simulink model "robot_simplified"  (R2021b)
settings: Solver=VariableStepAuto  StartTime=0.0  StopTime=11  RelTol=1e-3
model workspace: external: MATLAB File C:\Users\victo\Documents\MATLAB\CAD\STEP\ssl-robot\robot_simplified_DataFile.m (data not in the file)
values from neighbouring files (symbols this model uses):
  control =     [robot_simplified_DataFile.mat]
  g = 9.80665    [robot_simplified_DataFile.m]    (also in robot_simplified_parameters.m = -9.80665)
undefined symbols (not defined in the file or in its folder): DiscIntNeverNeededParam, field, kinematics, SamplingTime, smiData, tire, tkd, tki, tkp, wheel, X, Y, Z
libraries: sm_lib x722, nesl_utility x23, simulink x5, slpidlib x4, cstblocks x4, SignalEditorBlockLib x1, eeBldcCurrentController x1
(part 1 of 8)
settings Model: Creator=victo  LastModifiedBy=victo

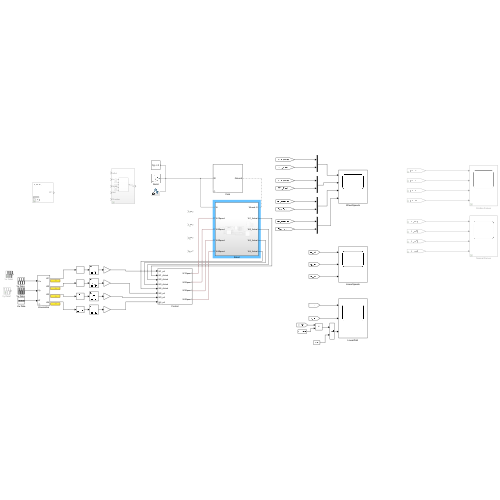
[thumbnail: Simulink's stored preview of the top-level diagram]
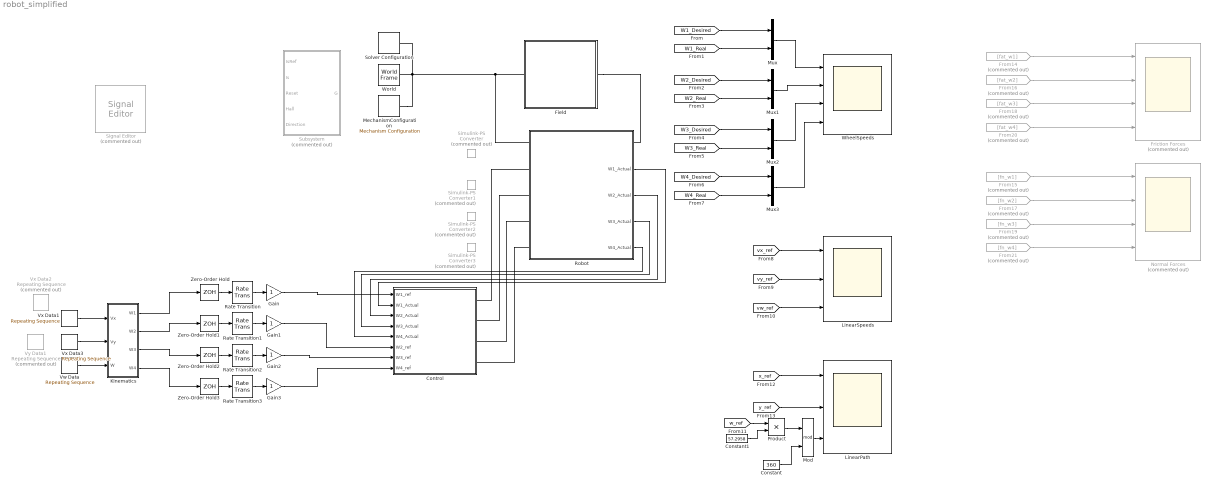
== system robot_simplified ==
  Constant : Constant  Value=360
  Constant1 : Constant  Value=57.2958
  Control : Subsystem  mask{T=SamplingTime, Kp=control.Kp, Ki=control.Ki, Ts=control.tf.Ts, df=control.tf.df, dm=control.tf.dm, FF=control.ff}
      mask prompts: T "Sampling Time"; Kp "Proportional"; Ki "Integral"
      mask DialogControl ControlParameters Prompt: Control Parameters
  Field : Subsystem  mask{fieldWidth=field.Width, fieldHeight=field.Height, fieldColor=field.Color}
      mask prompts: fieldWidth "Width(mm)"; fieldHeight "Height (mm)"; fieldColor "Color"
      mask DialogControl TabField Prompt: Field
  Friction Forces : Scope  Commented=on  NumInputPorts=4
  From14 : From  Commented=on  GotoTag=fat_w1
  From15 : From  Commented=on  GotoTag=fn_w1
  From16 : From  Commented=on  GotoTag=fat_w2
  From17 : From  Commented=on  GotoTag=fn_w2
  From18 : From  Commented=on  GotoTag=fat_w3
  From19 : From  Commented=on  GotoTag=fn_w3
  From20 : From  Commented=on  GotoTag=fat_w4
  From21 : From  Commented=on  GotoTag=fn_w4
  Gain{,1..3} (4 alike) : Gain
  Kinematics : Subsystem  mask{KinematicMatrix=kinematics.prod2}
      mask prompts: KinematicMatrix "Kinematics Function"
      mask DialogControl ParameterGroupVar0 Prompt: Kinematics Parameters
  LinearPath : Scope  NumInputPorts=3
  LinearSpeeds : Scope  NumInputPorts=3
  MechanismConfiguration : sm_lib/Utilities/Mechanism Configuration  UniformGravity=Constant  GravityVector="[0  0 -g]"  GravityUnits=m/s^2  LinearizationDelta=0.001  JointModeTransitionNonlinearIterations=2
  Mod : Math  Operator=mod  SaturateOnIntegerOverflow=on
  Mux{,1..3} (4 alike) : Mux  Inputs=2
  Normal Forces : Scope  Commented=on  NumInputPorts=4
  Product : Product
  Rate Transition : RateTransition  OutPortSampleTimeOpt=Inherit  OutPortSampleTime=0.002
  Rate Transition1 : RateTransition  OutPortSampleTimeOpt=Inherit  OutPortSampleTime=0.002
  Rate Transition2 : RateTransition  OutPortSampleTimeOpt=Inherit  OutPortSampleTime=0.01
  Rate Transition3 : RateTransition  OutPortSampleTimeOpt=Inherit  OutPortSampleTime=0.01
  Robot : Subsystem
      settings: PortSchema="{\"entries\":[{\"content\":{\"sides\":[{\"content\":{\"connectorIds\":[\"LConn1\",\"LConn2\",\"LConn3\",\"LConn4\",\"LConn5\"]},\"type\":\"ConnectorPlacement.EquallySpacedRectSide\",\"uuid\":\"253f09d1-5eeb-4b26-8135-d2db322c5f85\"},{\"content\":{\"connectorIds\":[\"RConn1\",\"Out1\",\"Out2\",\"Out3\",\"Out4\"],\"side\":\"RIGHT\"},\"type\":\"ConnectorPlacement.EquallySpacedRectSide\",\"uuid\":\"5e48723f-c100-4ab2-897b-63b213ce7996\"},{\"content\":{\"connectorIds\":[],\"side\":\"TOP\"},\"type\":\"ConnectorPlacement.EquallySpacedRectSide\",\"uuid\":\"88c9750e-929f-48a2-b612-d7f74cbee2f8\"}]},\"type\":\"ConnectorPlacement.EquallySpacedConnector\",\"uuid\":\"41f69800-7732-438a-91c0-e5f9fc926441\"}],\"packageUris\":[\"http://schema.mathworks.com/mf0/Connector/R2020b\"],\"version\":\"1.0\"}"
  Signal Editor : SignalEditorBlockLib/Signal Editor  Commented=on  FileName=Control_signals.mat  ActiveScenario=Scenario  ActiveSignal=W1  IsBus=off  OutputBusObjectStr=Bus: BusObject  SampleTime=0  ZeroCross=off  OutputAfterFinalValue=Holding final value  Unit=inherit  PreserveSignalName=on
  Simulink-PS Converter{,1..3} (4 alike) : nesl_utility/Simulink-PS Converter  Commented=on  PhysicalDomain=network_engine_domain  SubClassName=ps_input  LeftPortType=input  RightPortType=output  PseudoPeriodic=off  Frequencies=[]  NoiseDistribution=none  NoiseParameters=[]  Unit=1  AffineConversion=off  FilteringAndDerivatives=filter  SimscapeFilterOrder=2  InputFilterTimeConstant=0.001  UdotUserProvided=0
      settings: SourceProductBaseCode=PW,SS
  Solver Configuration : nesl_utility/Solver Configuration  PhysicalDomain=network_engine_domain  SubClassName=solver  LeftPortType=input  RightPortType=generic  Tones=[]  Harmonics=[]  SimulateNoise=off  Profile=off  UseLocalSampling=off  EnableSwitchedLinearOptims=on  FrequencyDomain=off  UseCCode=off  RelTol=0.001  AbsTol=1e-06  MinStep=1e-09  ToWorkspace=off  RevertToSquareIcSolve=off  NumHomotopyIterations=100  PhasorMode=off  PhasorModeNumHarmonics=1  DoDC=off  ResidualTolerance=1e-09  UseLocalSolver=off  LocalSolverChoice=NE_BACKWARD_EULER_ADVANCER  LocalSolverSampleTime=0.001  DoFixedCost=off  MaxNonlinIter=3  MaxModeIter=2  ComputeImpulses=off  ImpulseIterations=2  LinearAlgebra=Sparse  EquationFormulation=NE_TIME_EF  DelaysMemoryBudget=1024  AutomaticFiltering=on  FilteringTimeConstant=0.001  PartitionStorageMethod=AS_NEEDED  PartitionMemoryBudget=1024  PartitionMethod=ROBUST
      settings: SourceProductBaseCode=PW,SS
  Subsystem : Subsystem  Commented=on
  Vw Data : simulink/Sources/Repeating Sequence  rep_seq_t=[0 2 3 9.3 9.7 11]  rep_seq_y=[0 0 0 0 0 0]
  Vx Data1 : simulink/Sources/Repeating Sequence  rep_seq_t=[0 0.2 1 1.6 2.4 3.2 3.8 4.3 4.5 5.3 6 6.6 7 7.8 8.4 8.9 9.1 9.9 10.5 11]  rep_seq_y=[0 0 -0.75 0 0 0 0 0 0 0.75 0.75 0 0 0 0 0 0 -0.75 0 0]
  Vx Data2 : simulink/Sources/Repeating Sequence  Commented=on  rep_seq_t="[0 4.7  5.7 9.2 9.7 14.7 15.7 19.2 19.7 20]"  rep_seq_y=[0 0 -0.75 -0.75 0 0 0.75 0.75 0 0]
  Vx Data3 : simulink/Sources/Repeating Sequence  rep_seq_t=[0 0.2 1 1.6 2.3 3 3.8 4.1 4.3 4.5 5.3 6 6.6 6.7 7.4 8.2 8.5 8.9 9.1 9.9 10.5 11]  rep_seq_y=[0 0 -0.75 0 0 0.75 0.75 0 0 0 -0.75 -0.75 0 0 0.75 0.75 0 0 0 -0.75 0 0]
  Vy Data1 : simulink/Sources/Repeating Sequence  Commented=on  rep_seq_t=[0 0.2 1.2 3.7 4.2 10.2 11.2 13.7 14.2 20]  rep_seq_y=[0 0 0.75 0.75 0 0 -0.75 -0.75 0 0]
  WheelSpeeds : Scope  NumInputPorts=4
  World : sm_lib/Frames and Transforms/World Frame
  Zero-Order Hold{,1..3} (4 alike) : ZeroOrderHold  SampleTime=0.002
  wires:
  Mux/1 -> WheelSpeeds/1
  Robot/2(W2_Actual) -> Control/3(W2_Actual)
  Robot/3(W3_Actual) -> Control/4(W3_Actual)
  Robot/4(W4_Actual) -> Control/5(W4_Actual)
  [W2_Desired] -> Mux1/1
  [W2_Real] -> Mux1/2
  [W3_Desired] -> Mux2/1
  [W3_Real] -> Mux2/2
  [W4_Desired] -> Mux3/1
  [W4_Real] -> Mux3/2
  Rate Transition/1 -> Gain/1
  Zero-Order Hold/1 -> Rate Transition/1
  Zero-Order Hold1/1 -> Rate Transition1/1
  Rate Transition1/1 -> Gain1/1
  Zero-Order Hold2/1 -> Rate Transition2/1
  Rate Transition2/1 -> Gain2/1
  Zero-Order Hold3/1 -> Rate Transition3/1
  Rate Transition3/1 -> Gain3/1
  Gain/1 -> Control/1(W1_ref)
  Robot/1(W1_Actual) -> Control/2(W1_Actual)
  Gain1/1 -> Control/6(W2_ref)
  Gain2/1 -> Control/7(W3_ref)
  Gain3/1 -> Control/8(W4_ref)
  [W1_Real] -> Mux/2
  [W1_Desired] -> Mux/1
  Mux1/1 -> WheelSpeeds/2
  Mux2/1 -> WheelSpeeds/3
  Mux3/1 -> WheelSpeeds/4
  [vx_ref] -> LinearSpeeds/1
  [vy_ref] -> LinearSpeeds/2
  [vw_ref] -> LinearSpeeds/3
  [x_ref] -> LinearPath/1
  [y_ref] -> LinearPath/2
  Constant/1 -> Mod/2
  Mod/1 -> LinearPath/3
  [w_ref] -> Product/1
  Constant1/1 -> Product/2
  Product/1 -> Mod/1
  Vw Data/1 -> Kinematics/3(W)
  Kinematics/4(W4) -> Zero-Order Hold3/1
  Kinematics/1(W1) -> Zero-Order Hold/1
  Kinematics/2(W2) -> Zero-Order Hold1/1
  Kinematics/3(W3) -> Zero-Order Hold2/1
  Vx Data3/1 -> Kinematics/2(Vy)
  Vx Data1/1 -> Kinematics/1(Vx)
  From14/1 -> Friction Forces/1
  From18/1 -> Friction Forces/3
  From17/1 -> Normal Forces/2
  From20/1 -> Friction Forces/4
  From19/1 -> Normal Forces/3
  From16/1 -> Friction Forces/2
  From21/1 -> Normal Forces/4
  From15/1 -> Normal Forces/1
  connections:
  MechanismConfiguration/RConn1 -- Field/LConn1 -- Robot/LConn1 -- Solver Configuration/RConn1 -- World/RConn1
  Field/RConn1 -- Robot/RConn1
  Robot/LConn2 -- Control/RConn1
  Robot/LConn3 -- Control/RConn2
  Robot/LConn4 -- Control/RConn3
  Robot/LConn5 -- Control/RConn4

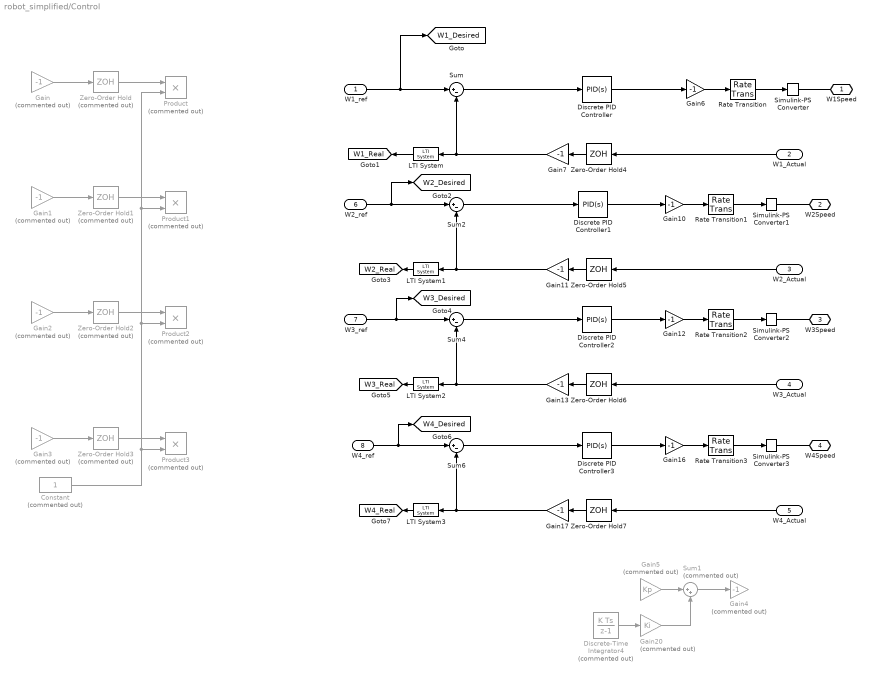
== system robot_simplified/Control ==
  W1_ref : Inport
  W1_Actual : Inport  Port=2
  W2_Actual : Inport  Port=3
  W3_Actual : Inport  Port=4
  W4_Actual : Inport  Port=5
  W2_ref : Inport  Port=6
  W3_ref : Inport  Port=7
  W4_ref : Inport  Port=8
  Constant : Constant  Commented=on
  Discrete PID Controller : slpidlib/PID Controller  Controller=PID  Form=Parallel  TimeDomain=Continuous-time  UseExternalTs=off  SampleTime=-1  IntegratorMethod=Forward Euler  FilterMethod=Forward Euler  ControllerParametersSource=internal  P=tkp  I=tki  D=tkd  UseFilter=on  N=8276.77127710328  TunerSelectOption=Transfer Function Based (PID Tuner App)  InitialConditionSource=internal  InitialConditionForIntegrator=0  InitialConditionForFilter=0  DifferentiatorICPrevScaledInput=0  ExternalReset=none  TrackingMode=off  Kt=1  LimitOutput=off  SatLimitsSource=internal  UpperSaturationLimit=2527  LowerSaturationLimit=-2527  LinearizeAsGain=off  AntiWindupMode=clamping  Kb=1  POutMin=[]  POutMax=[]  IOutMin=[]  IOutMax=[]  DOutMin=[]  DOutMax=[]  NOutMin=[]  NOutMax=[]  SumOutMin=[]  SumOutMax=[]  SaturationOutMin=[]  SaturationOutMax=[]  PParamMin=[]  PParamMax=[]  IParamMin=[]  IParamMax=[]  DParamMin=[]  DParamMax=[]  NParamMin=[]  NParamMax=[]  KbParamMin=[]  KbParamMax=[]  KtParamMin=[]  KtParamMax=[]  KbOutMin=[]  KbOutMax=[]  KtOutMin=[]  KtOutMax=[]  IntegratorOutMin=[]  IntegratorOutMax=[]  FilterOutMin=[]  FilterOutMax=[]  SumI1OutMin=[]  SumI1OutMax=[]  SumI2OutMin=[]  SumI2OutMax=[]  SumI3OutMin=[]  SumI3OutMax=[]  SumI4OutMin=[]  SumI4OutMax=[]  SumDOutMin=[]  SumDOutMax=[]  DifferentiatorOutMin=[]  DifferentiatorOutMax=[]  FilterDiffOutCoefMin=[]  FilterDiffOutCoefMax=[]  ReciprocalOutMin=[]  ReciprocalOutMax=[]  SumDenOutMin=[]  SumDenOutMax=[]  SumNumOutMin=[]  SumNumOutMax=[]  DivideOutMin=[]  DivideOutMax=[]  UdiffTsProdOutMin=[]  UdiffTsProdOutMax=[]  NTsProdOutMin=[]  NTsProdOutMax=[]  UintegralTsProdOutMin=[]  UintegralTsProdOutMax=[]  UngainTsProdOutMin=[]  UngainTsProdOutMax=[]  IntegratorContinuousStateAttributes=''  IntegratorStateMustResolveToSignalObject=off  IntegratorRTWStateStorageClass=Auto  FilterContinuousStateAttributes=''  FilterStateMustResolveToSignalObject=off  FilterRTWStateStorageClass=Auto  ParallelPVariant=InternalParameters  IdealPVariant=Disabled  IVariant=InternalParameters  DVariant=InternalParameters  IntegratorVariant=Continuous  SatVariant=Disabled  AWVariant=Passthrough  PCopyVariant=Disabled  TRVariant=Disabled  FdbkBlocksVariant=Forward  IdealPFdbkVariant=Disabled  SatFdbkVariant=Disabled  DerivativeFilterVariant=ContFilter  NVariant=InternalParameters  NCopyVariant=Disabled  FilterICVariant=InternalICsFilter  IntegratorICVariant=InternalICs  ExternalResetVariant=Disabled  TRSumVariant=Passthrough  SumFdbkVariant=Disabled  SumVariant=Sum_PID  TsampFilterVariant=InternalTs  TsampNgainVariant=Passthrough  TsampIntegralVariant=Passthrough  ExternalSaturationOutDataTypeStr=Inherit: Same as second input
  Discrete PID Controller1 : slpidlib/PID Controller  Controller=PID  Form=Parallel  TimeDomain=Continuous-time  UseExternalTs=off  SampleTime=0.01  IntegratorMethod=Forward Euler  FilterMethod=Forward Euler  ControllerParametersSource=internal  P=tkp  I=tki  D=tkd  UseFilter=on  N=7595.87594615657  TunerSelectOption=Transfer Function Based (PID Tuner App)  InitialConditionSource=internal  InitialConditionForIntegrator=0  InitialConditionForFilter=0  DifferentiatorICPrevScaledInput=0  ExternalReset=none  TrackingMode=off  Kt=1  LimitOutput=off  SatLimitsSource=internal  UpperSaturationLimit=2527  LowerSaturationLimit=-2527  LinearizeAsGain=off  AntiWindupMode=clamping  Kb=1  POutMin=[]  POutMax=[]  IOutMin=[]  IOutMax=[]  DOutMin=[]  DOutMax=[]  NOutMin=[]  NOutMax=[]  SumOutMin=[]  SumOutMax=[]  SaturationOutMin=[]  SaturationOutMax=[]  PParamMin=[]  PParamMax=[]  IParamMin=[]  IParamMax=[]  DParamMin=[]  DParamMax=[]  NParamMin=[]  NParamMax=[]  KbParamMin=[]  KbParamMax=[]  KtParamMin=[]  KtParamMax=[]  KbOutMin=[]  KbOutMax=[]  KtOutMin=[]  KtOutMax=[]  IntegratorOutMin=[]  IntegratorOutMax=[]  FilterOutMin=[]  FilterOutMax=[]  SumI1OutMin=[]  SumI1OutMax=[]  SumI2OutMin=[]  SumI2OutMax=[]  SumI3OutMin=[]  SumI3OutMax=[]  SumI4OutMin=[]  SumI4OutMax=[]  SumDOutMin=[]  SumDOutMax=[]  DifferentiatorOutMin=[]  DifferentiatorOutMax=[]  FilterDiffOutCoefMin=[]  FilterDiffOutCoefMax=[]  ReciprocalOutMin=[]  ReciprocalOutMax=[]  SumDenOutMin=[]  SumDenOutMax=[]  SumNumOutMin=[]  SumNumOutMax=[]  DivideOutMin=[]  DivideOutMax=[]  UdiffTsProdOutMin=[]  UdiffTsProdOutMax=[]  NTsProdOutMin=[]  NTsProdOutMax=[]  UintegralTsProdOutMin=[]  UintegralTsProdOutMax=[]  UngainTsProdOutMin=[]  UngainTsProdOutMax=[]  IntegratorContinuousStateAttributes=''  IntegratorStateMustResolveToSignalObject=off  IntegratorRTWStateStorageClass=Auto  FilterContinuousStateAttributes=''  FilterStateMustResolveToSignalObject=off  FilterRTWStateStorageClass=Auto  ParallelPVariant=InternalParameters  IdealPVariant=Disabled  IVariant=InternalParameters  DVariant=InternalParameters  IntegratorVariant=Continuous  SatVariant=Disabled  AWVariant=Passthrough  PCopyVariant=Disabled  TRVariant=Disabled  FdbkBlocksVariant=Forward  IdealPFdbkVariant=Disabled  SatFdbkVariant=Disabled  DerivativeFilterVariant=ContFilter  NVariant=InternalParameters  NCopyVariant=Disabled  FilterICVariant=InternalICsFilter  IntegratorICVariant=InternalICs  ExternalResetVariant=Disabled  TRSumVariant=Passthrough  SumFdbkVariant=Disabled  SumVariant=Sum_PID  TsampFilterVariant=InternalTs  TsampNgainVariant=Passthrough  TsampIntegralVariant=Passthrough  ExternalSaturationOutDataTypeStr=Inherit: Same as second input
  Discrete PID Controller2 : slpidlib/PID Controller  Controller=PID  Form=Parallel  TimeDomain=Continuous-time  UseExternalTs=off  SampleTime=0.01  IntegratorMethod=Forward Euler  FilterMethod=Forward Euler  ControllerParametersSource=internal  P=tkp  I=tki  D=tkd  UseFilter=on  N=7595.87594615657  TunerSelectOption=Transfer Function Based (PID Tuner App)  InitialConditionSource=internal  InitialConditionForIntegrator=0  InitialConditionForFilter=0  DifferentiatorICPrevScaledInput=0  ExternalReset=none  TrackingMode=off  Kt=1  LimitOutput=off  SatLimitsSource=internal  UpperSaturationLimit=2527  LowerSaturationLimit=-2527  LinearizeAsGain=off  AntiWindupMode=clamping  Kb=1  POutMin=[]  POutMax=[]  IOutMin=[]  IOutMax=[]  DOutMin=[]  DOutMax=[]  NOutMin=[]  NOutMax=[]  SumOutMin=[]  SumOutMax=[]  SaturationOutMin=[]  SaturationOutMax=[]  PParamMin=[]  PParamMax=[]  IParamMin=[]  IParamMax=[]  DParamMin=[]  DParamMax=[]  NParamMin=[]  NParamMax=[]  KbParamMin=[]  KbParamMax=[]  KtParamMin=[]  KtParamMax=[]  KbOutMin=[]  KbOutMax=[]  KtOutMin=[]  KtOutMax=[]  IntegratorOutMin=[]  IntegratorOutMax=[]  FilterOutMin=[]  FilterOutMax=[]  SumI1OutMin=[]  SumI1OutMax=[]  SumI2OutMin=[]  SumI2OutMax=[]  SumI3OutMin=[]  SumI3OutMax=[]  SumI4OutMin=[]  SumI4OutMax=[]  SumDOutMin=[]  SumDOutMax=[]  DifferentiatorOutMin=[]  DifferentiatorOutMax=[]  FilterDiffOutCoefMin=[]  FilterDiffOutCoefMax=[]  ReciprocalOutMin=[]  ReciprocalOutMax=[]  SumDenOutMin=[]  SumDenOutMax=[]  SumNumOutMin=[]  SumNumOutMax=[]  DivideOutMin=[]  DivideOutMax=[]  UdiffTsProdOutMin=[]  UdiffTsProdOutMax=[]  NTsProdOutMin=[]  NTsProdOutMax=[]  UintegralTsProdOutMin=[]  UintegralTsProdOutMax=[]  UngainTsProdOutMin=[]  UngainTsProdOutMax=[]  IntegratorContinuousStateAttributes=''  IntegratorStateMustResolveToSignalObject=off  IntegratorRTWStateStorageClass=Auto  FilterContinuousStateAttributes=''  FilterStateMustResolveToSignalObject=off  FilterRTWStateStorageClass=Auto  ParallelPVariant=InternalParameters  IdealPVariant=Disabled  IVariant=InternalParameters  DVariant=InternalParameters  IntegratorVariant=Continuous  SatVariant=Disabled  AWVariant=Passthrough  PCopyVariant=Disabled  TRVariant=Disabled  FdbkBlocksVariant=Forward  IdealPFdbkVariant=Disabled  SatFdbkVariant=Disabled  DerivativeFilterVariant=ContFilter  NVariant=InternalParameters  NCopyVariant=Disabled  FilterICVariant=InternalICsFilter  IntegratorICVariant=InternalICs  ExternalResetVariant=Disabled  TRSumVariant=Passthrough  SumFdbkVariant=Disabled  SumVariant=Sum_PID  TsampFilterVariant=InternalTs  TsampNgainVariant=Passthrough  TsampIntegralVariant=Passthrough  ExternalSaturationOutDataTypeStr=Inherit: Same as second input
  Discrete PID Controller3 : slpidlib/PID Controller  Controller=PID  Form=Parallel  TimeDomain=Continuous-time  UseExternalTs=off  SampleTime=0.01  IntegratorMethod=Forward Euler  FilterMethod=Forward Euler  ControllerParametersSource=internal  P=tkp  I=tki  D=tkd  UseFilter=on  N=7595.87594615657  TunerSelectOption=Transfer Function Based (PID Tuner App)  InitialConditionSource=internal  InitialConditionForIntegrator=0  InitialConditionForFilter=0  DifferentiatorICPrevScaledInput=0  ExternalReset=none  TrackingMode=off  Kt=1  LimitOutput=off  SatLimitsSource=internal  UpperSaturationLimit=2527  LowerSaturationLimit=-2527  LinearizeAsGain=off  AntiWindupMode=clamping  Kb=1  POutMin=[]  POutMax=[]  IOutMin=[]  IOutMax=[]  DOutMin=[]  DOutMax=[]  NOutMin=[]  NOutMax=[]  SumOutMin=[]  SumOutMax=[]  SaturationOutMin=[]  SaturationOutMax=[]  PParamMin=[]  PParamMax=[]  IParamMin=[]  IParamMax=[]  DParamMin=[]  DParamMax=[]  NParamMin=[]  NParamMax=[]  KbParamMin=[]  KbParamMax=[]  KtParamMin=[]  KtParamMax=[]  KbOutMin=[]  KbOutMax=[]  KtOutMin=[]  KtOutMax=[]  IntegratorOutMin=[]  IntegratorOutMax=[]  FilterOutMin=[]  FilterOutMax=[]  SumI1OutMin=[]  SumI1OutMax=[]  SumI2OutMin=[]  SumI2OutMax=[]  SumI3OutMin=[]  SumI3OutMax=[]  SumI4OutMin=[]  SumI4OutMax=[]  SumDOutMin=[]  SumDOutMax=[]  DifferentiatorOutMin=[]  DifferentiatorOutMax=[]  FilterDiffOutCoefMin=[]  FilterDiffOutCoefMax=[]  ReciprocalOutMin=[]  ReciprocalOutMax=[]  SumDenOutMin=[]  SumDenOutMax=[]  SumNumOutMin=[]  SumNumOutMax=[]  DivideOutMin=[]  DivideOutMax=[]  UdiffTsProdOutMin=[]  UdiffTsProdOutMax=[]  NTsProdOutMin=[]  NTsProdOutMax=[]  UintegralTsProdOutMin=[]  UintegralTsProdOutMax=[]  UngainTsProdOutMin=[]  UngainTsProdOutMax=[]  IntegratorContinuousStateAttributes=''  IntegratorStateMustResolveToSignalObject=off  IntegratorRTWStateStorageClass=Auto  FilterContinuousStateAttributes=''  FilterStateMustResolveToSignalObject=off  FilterRTWStateStorageClass=Auto  ParallelPVariant=InternalParameters  IdealPVariant=Disabled  IVariant=InternalParameters  DVariant=InternalParameters  IntegratorVariant=Continuous  SatVariant=Disabled  AWVariant=Passthrough  PCopyVariant=Disabled  TRVariant=Disabled  FdbkBlocksVariant=Forward  IdealPFdbkVariant=Disabled  SatFdbkVariant=Disabled  DerivativeFilterVariant=ContFilter  NVariant=InternalParameters  NCopyVariant=Disabled  FilterICVariant=InternalICsFilter  IntegratorICVariant=InternalICs  ExternalResetVariant=Disabled  TRSumVariant=Passthrough  SumFdbkVariant=Disabled  SumVariant=Sum_PID  TsampFilterVariant=InternalTs  TsampNgainVariant=Passthrough  TsampIntegralVariant=Passthrough  ExternalSaturationOutDataTypeStr=Inherit: Same as second input
  Discrete-Time Integrator4 : DiscreteIntegrator  Commented=on  SampleTime=-1  ICPrevOutput=DiscIntNeverNeededParam  ICPrevScaledInput=DiscIntNeverNeededParam
  Gain{,1..4} (5 alike) : Gain  Commented=on  Gain=-1
  Gain{6..7,10..13,16..17} (8 alike) : Gain  Gain=-1
  Gain20 : Gain  Commented=on  Gain=Ki
  Gain5 : Gain  Commented=on  Gain=Kp
  LTI System{,1..3} (4 alike) : cstblocks/LTI System  sys=FF  IC=[]
  Product{,1..3} (4 alike) : Product  Commented=on
  Rate Transition : RateTransition  OutPortSampleTimeOpt=Inherit  OutPortSampleTime=0.01
  Rate Transition1 : RateTransition  OutPortSampleTimeOpt=Inherit
  Rate Transition2 : RateTransition  OutPortSampleTimeOpt=Inherit  OutPortSampleTime=0.01
  Rate Transition3 : RateTransition  OutPortSampleTimeOpt=Inherit  OutPortSampleTime=0.01
  Simulink-PS Converter{,1..3} (4 alike) : nesl_utility/Simulink-PS Converter  PhysicalDomain=network_engine_domain  SubClassName=ps_input  LeftPortType=input  RightPortType=output  PseudoPeriodic=off  Frequencies=[]  NoiseDistribution=none  NoiseParameters=[]  Unit=1  AffineConversion=off  FilteringAndDerivatives=filter  SimscapeFilterOrder=2  InputFilterTimeConstant=0.01  UdotUserProvided=0
      settings: SourceProductBaseCode=PW,SS
  Sum{,2,4,6} (4 alike) : Sum  Inputs=|+-
  Sum1 : Sum  Commented=on  Inputs=|++
  Zero-Order Hold{,1..3} (4 alike) : ZeroOrderHold  Commented=on  SampleTime=T
  Zero-Order Hold4 : ZeroOrderHold  SampleTime=-1
  Zero-Order Hold5 : ZeroOrderHold  SampleTime=0.01
  Zero-Order Hold6 : ZeroOrderHold  SampleTime=-1
  Zero-Order Hold7 : ZeroOrderHold  SampleTime=-1
  W1Speed : PMIOPort  Side=Right
  W2Speed : PMIOPort  Port=2  Side=Right
  W3Speed : PMIOPort  Port=3  Side=Right
  W4Speed : PMIOPort  Port=4  Side=Right
  tag scope: W1_Desired=global, W1_Real=global, W2_Desired=global, W2_Real=global, W3_Desired=global, W3_Real=global, W4_Desired=global, W4_Real=global
  wires:
  Gain/1 -> Zero-Order Hold/1
  Gain1/1 -> Zero-Order Hold1/1
  Gain2/1 -> Zero-Order Hold2/1
  Gain3/1 -> Zero-Order Hold3/1
  Zero-Order Hold/1 -> Product/1
  Constant/1 -> Product3/2, Product2/2, Product1/2, Product/2
  Zero-Order Hold1/1 -> Product1/1
  Zero-Order Hold2/1 -> Product2/1
  Zero-Order Hold3/1 -> Product3/1
  Rate Transition/1 -> Simulink-PS Converter/1
  Gain6/1 -> Rate Transition/1
  Discrete PID Controller/1 -> Gain6/1
  Zero-Order Hold4/1 -> Gain7/1
  W1_Actual/1 -> Zero-Order Hold4/1
  Gain7/1 -> LTI System/1, Sum/2
  Gain11/1 -> Sum2/2, LTI System1/1
  Sum2/1 -> Discrete PID Controller1/1
  W2_Actual/1 -> Zero-Order Hold5/1
  Gain10/1 -> Rate Transition1/1
  Zero-Order Hold5/1 -> Gain11/1
  Rate Transition1/1 -> Simulink-PS Converter1/1
  LTI System1/1 -> [W2_Real]
  Rate Transition2/1 -> Simulink-PS Converter2/1
  LTI System2/1 -> [W3_Real]
  Gain12/1 -> Rate Transition2/1
  Zero-Order Hold6/1 -> Gain13/1
  Sum4/1 -> Discrete PID Controller2/1
  Gain13/1 -> Sum4/2, LTI System2/1
  W3_Actual/1 -> Zero-Order Hold6/1
  W4_Actual/1 -> Zero-Order Hold7/1
  Gain17/1 -> Sum6/2, LTI System3/1
  Sum6/1 -> Discrete PID Controller3/1
  Zero-Order Hold7/1 -> Gain17/1
  LTI System3/1 -> [W4_Real]
  Rate Transition3/1 -> Simulink-PS Converter3/1
  Gain16/1 -> Rate Transition3/1
  Discrete PID Controller3/1 -> Gain16/1
  W1_ref/1 -> [W1_Desired], Sum/1
  W2_ref/1 -> [W2_Desired], Sum2/1
  W3_ref/1 -> [W3_Desired], Sum4/1
  W4_ref/1 -> [W4_Desired], Sum6/1
  Sum/1 -> Discrete PID Controller/1
  Gain5/1 -> Sum1/1
  Sum1/1 -> Gain4/1
  Gain20/1 -> Sum1/2
  Discrete-Time Integrator4/1 -> Gain20/1
  Discrete PID Controller1/1 -> Gain10/1
  Discrete PID Controller2/1 -> Gain12/1
  LTI System/1 -> [W1_Real]
  connections:
  Simulink-PS Converter/RConn1 -- W1Speed/RConn1
  Simulink-PS Converter1/RConn1 -- W2Speed/RConn1
  Simulink-PS Converter2/RConn1 -- W3Speed/RConn1
  Simulink-PS Converter3/RConn1 -- W4Speed/RConn1

== system robot_simplified/Field ==
  Field objects : Subsystem  mask{HorizontalWallsWidth=field.walls.Width1, HorizontalWallsLength=field.walls.Length1, HorizontalWallsHeight=field.walls.Height1, VerticalWallsWidth=field.walls.Width2, VerticalWallsLength=field.walls.Length2, VerticalWallsHeight=field.walls.Height2, HorizontalWallsAxis=field.walls.axis1, HorizontalWallsTransform=field.walls.transform1, HorizontalWallsAxis2=field.walls.axis2, HorizontalWallsTransform2=field.walls.transform2, HorizontalWallsAxis3=field.walls.axis3, HorizontalWallsTransform3=field.walls.transform3, HorizontalWallsAxis4=field.walls.axis3, HorizontalWallsTransform4=field.walls.transform4, GoalLatWallsWidth=field.goals.Width1, GoalLatWallsLength=field.goals.Length1, GoalLatWallsHeight=field.goals.Height1, GoalBackWallsWidth=field.goals.Width2, GoalBackWallsLength=field.goals.Length2, GoalBackWallsHeight=field.goals.Height2, GoalLatAxis1=field.goals.axis1, GoalLatAxis2=field.goals.axis2, GoalLatTransform1=field.goals.transform1, GoalLatTransform2=field.goals.transform2, GoalLatTransform3=field.goals.transform3, GoalLatTransform4=field.goals.transform4, GoalBackTransform1=field.goals.transform5, GoalBackTransform2=field.goals.transform6, HorizontalFieldLineWidth=field.lines.Width2, HorizontalFieldLineLength=field.lines.Length2, HorizontalFieldLineHeight=field.lines.Height2, VerticalFieldLineWidth=field.lines.Width1, VerticalFieldLineLength=field.lines.Length1, VerticalFieldLineHeight=field.lines.Height1, HorizontalGoalLineWidth=field.lines.Width2, HorizontalGoalLineLength=field.lines.Length2, HorizontalGoalLineHeight=field.lines.Height2, VerticalGoalLineWidth=field.lines.Width1, VerticalGoalLineLength=field.lines.Length1, VerticalGoalLineHeight=field.lines.Height2, MidLineCircleInternalDiameter=field.lines.Radius1, MidLineCircleExternalDiameter=field.lines.Radius2, MidLineCircleHeight=field.lines.Height, HorizontalFieldLineTransform1=field.lines.transform1, HorizontalFieldLineTransform2=field.lines.transform2, VerticalFieldLineTransform1=field.lines.transform3, VerticalFieldLineTransform2=field.lines.transform4}
      mask prompts: HorizontalWallsWidth "Horizontal Walls Width"; HorizontalWallsLength "Horizontal Walls Length"; HorizontalWallsHeight "Horizontal Walls Height"; VerticalWallsWidth "Vertical Walls Width"; VerticalWallsLength "Vertical Walls Length"; VerticalWallsHeight "Vertical Walls Height"; HorizontalWallsAxis "Horizontal Walls Axis"; HorizontalWallsTransform "Horizontal Walls Transform"; HorizontalWallsAxis2 "Horiontal Walls Axis2"; HorizontalWallsTransform2 "Horizontal Walls Transform2"; HorizontalWallsAxis3 "Horiontal Walls Axis3"; HorizontalWallsTransform3 "Horizontal Walls Transform3"; HorizontalWallsAxis4 "Horiontal Walls Axis4"; HorizontalWallsTransform4 "Horizontal Walls Transform4"; GoalLatWallsWidth "Goal Lateral Walls Width"; GoalLatWallsLength "Goal Lateral Walls Length"; GoalLatWallsHeight "Goal Lateral Walls Height"; GoalLatAxis1 "Goal Lateral Axis1"; GoalLatAxis2 "Goal Lateral Axis2"; GoalLatTransform1 "Goal Lateral Transform1"; GoalLatTransform2 "Goal Lateral Transform2"; GoalLatTransform3 "Goal Lateral Transform3"; GoalLatTransform4 "Goal Lateral Transform4"; GoalBackTransform1 "Goal Back Transform1"; GoalBackTransform2 "Goal Back Transform2"; HorizontalFieldLineWidth "Horizontal Field Line Width"; HorizontalFieldLineLength "Horizontal Field Line Length"; HorizontalFieldLineHeight "Horizontal Field Line Height"; VerticalFieldLineWidth "Vertical Field Line Width"; VerticalFieldLineLength "Vertical Field Line Length"; VerticalFieldLineHeight "Vertical Field Line Height"; HorizontalGoalLineWidth "Horizontal Goal Line Width"; HorizontalGoalLineLength "Horizontal Goal Line Length"; HorizontalGoalLineHeight "Horizontal Goal Line Height"; VerticalGoalLineWidth "Vertical Goal Line Width"; VerticalGoalLineLength "Vertical Goal Line Length"; VerticalGoalLineHeight "Vertical Goal Line Height"; MidLineCircleInternalDiameter "Mid Line Circle Internal Diameter"; MidLineCircleExternalDiameter "Mid Line Circle External Diameter"; MidLineCircleHeight "Mid Line Circle Height"; HorizontalFieldLineTransform1 "Horizontal Field Line Transform1"; HorizontalFieldLineTransform2 "Horizontal Field Line Transform2"; VerticalFieldLineTransform1 "Vertical Field Line Transform1"
      mask DialogControl ParameterGroupVar Prompt: Wall Parameters
      mask DialogControl ParameterGroupVar01 Prompt: Goal Parameters
      mask DialogControl ParameterGroupVar02 Prompt: Field Line Parameters
  Ground Alignment : sm_lib/Frames and Transforms/Rigid Transform  TranslationMethod=Cartesian  TranslationStandardOffset=0  TranslationLengthUnit=mm  TranslationStandardAxis=+Z  TranslationCartesianOffset=[0 0 -9.5]  TranslationROffset=0  TranslationROffsetUnits=m  TranslationZOffset=0  TranslationZOffsetUnits=m  TranslationThetaOffset=0  TranslationThetaOffsetUnits=deg  RotationMethod=None  RotationAngleUnits=deg  RotationStandardAxis=+X  RotationAngle=-90  RotationArbitraryAxis=[0 0 1]  FollAlignAxisA=+X  BaseAlignAxisA=+Y  FollAlignAxisB=+Y  BaseAlignAxisB=+Z  RotationSequenceAxes=FollowerAxes  RotationSequence=XYX  RotationSequenceAngles=[0 0 0]  RotationSequenceAnglesUnits=deg  RotationMatrix=[1 0 0; 0 1 0; 0 0 1]
  Infinite Plane : sm_lib/Curves and Surfaces/Infinite Plane  GraphicType=Rectangle  GraphicPlaneWidth=fieldWidth  GraphicPlaneWidthUnits=mm  GraphicPlaneHeight=fieldHeight  GraphicPlaneHeightUnits=mm  GraphicVisPropType=SimpleVisualProperties  GraphicDiffuseColor=fieldColor  GraphicOpacity=1  GraphicSpecularColor=[0.5 0.5 0.5 1.0]  GraphicAmbientColor=[0.15 0.15 0.15 1.0]  GraphicEmissiveColor=[0.0 0.0 0.0 1.0]  GraphicShininess=75
  W : PMIOPort  Side=Left
  Ground : PMIOPort  Port=2  Side=Right
  connections:
  Infinite Plane/RConn1 -- Ground/RConn1
  W/RConn1 -- Field objects/RConn1 -- Ground Alignment/LConn1
  Ground Alignment/RConn1 -- Infinite Plane/LConn1

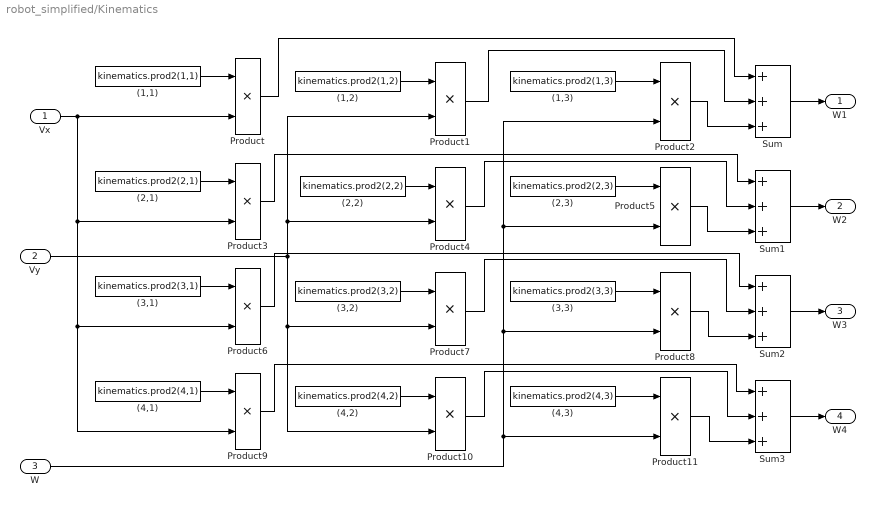
== system robot_simplified/Kinematics ==
  Vx : Inport
  Vy : Inport  Port=2
  W : Inport  Port=3
  (1,1) : Constant  Value=kinematics.prod2(1,1)
  (1,2) : Constant  Value=kinematics.prod2(1,2)
  (1,3) : Constant  Value=kinematics.prod2(1,3)
  (2,1) : Constant  Value=kinematics.prod2(2,1)
  (2,2) : Constant  Value=kinematics.prod2(2,2)
  (2,3) : Constant  Value=kinematics.prod2(2,3)
  (3,1) : Constant  Value=kinematics.prod2(3,1)
  (3,2) : Constant  Value=kinematics.prod2(3,2)
  (3,3) : Constant  Value=kinematics.prod2(3,3)
  (4,1) : Constant  Value=kinematics.prod2(4,1)
  (4,2) : Constant  Value=kinematics.prod2(4,2)
  (4,3) : Constant  Value=kinematics.prod2(4,3)
  Product{,1..11} (12 alike) : Product
  Sum{,1..3} (4 alike) : Sum  Inputs=+++
  W1 : Outport
  W2 : Outport  Port=2
  W3 : Outport  Port=3
  W4 : Outport  Port=4
  wires:
  (1,1)/1 -> Product/1
  Vx/1 -> Product9/2, Product6/2, Product3/2, Product/2
  (1,2)/1 -> Product1/1
  Vy/1 -> Product1/2, Product4/2, Product10/2, Product7/2
  (1,3)/1 -> Product2/1
  W/1 -> Product11/2, Product5/2, Product2/2, Product8/2
  Sum/1 -> W1/1
  Product/1 -> Sum/1
  Product1/1 -> Sum/2
  Product2/1 -> Sum/3
  (2,1)/1 -> Product3/1
  (2,2)/1 -> Product4/1
  (2,3)/1 -> Product5/1
  Product3/1 -> Sum1/1
  Product4/1 -> Sum1/2
  Product5/1 -> Sum1/3
  Sum1/1 -> W2/1
  (3,1)/1 -> Product6/1
  (3,2)/1 -> Product7/1
  (3,3)/1 -> Product8/1
  Product6/1 -> Sum2/1
  Product7/1 -> Sum2/2
  Product8/1 -> Sum2/3
  Sum2/1 -> W3/1
  (4,1)/1 -> Product9/1
  (4,2)/1 -> Product10/1
  (4,3)/1 -> Product11/1
  Product9/1 -> Sum3/1
  Product10/1 -> Sum3/2
  Product11/1 -> Sum3/3
  Sum3/1 -> W4/1

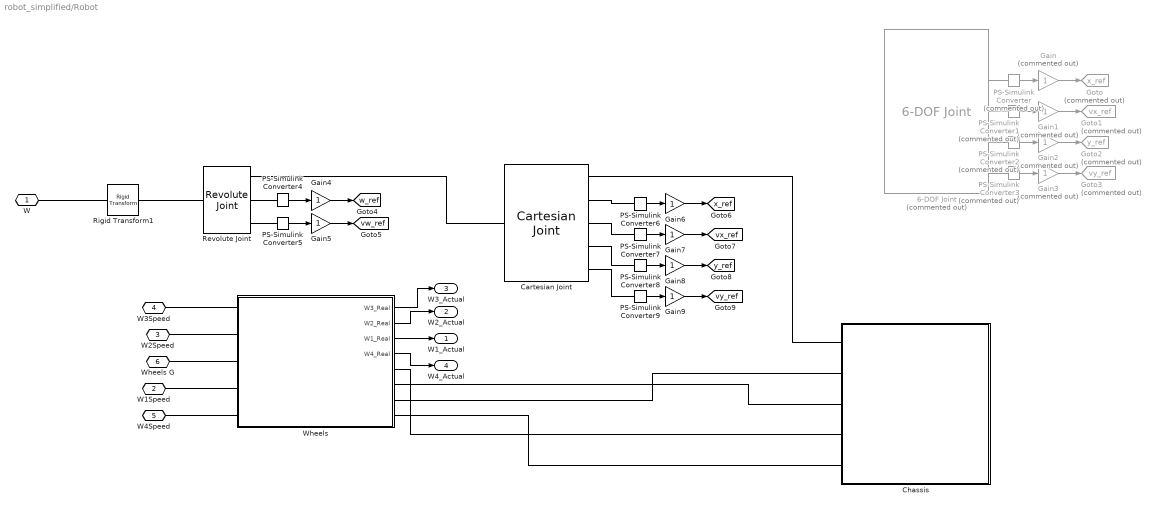
== system robot_simplified/Robot ==
  6-DOF Joint : sm_lib/Joints/6-DOF Joint  Commented=on  JointMode=Normal  SenseConstraintForce=off  SenseConstraintForceX=off  SenseConstraintForceY=off  SenseConstraintForceZ=off  SenseConstraintTorque=off  SenseConstraintTorqueX=off  SenseConstraintTorqueY=off  SenseConstraintTorqueZ=off  SenseTotalForce=off  SenseTotalForceX=off  SenseTotalForceY=off  SenseTotalForceZ=off  SenseTotalTorque=off  SenseTotalTorqueX=off  SenseTotalTorqueY=off  SenseTotalTorqueZ=off  CompositeWrenchDir=FollowerOnBase  CompositeWrenchFrame=BaseFrame  PxEquilibriumPosition=0  PxEquilibriumPositionUnits=m  PxSpringStiffness=0  PxSpringStiffnessUnits=N/m  PxDampingCoefficient=1e-3  PxDampingCoefficientUnits=N/(m/s)  PxTorqueActuationMode=NoTorque  PxMotionActuationMode=ComputedMotion  PxSensePosition=on  PxSenseVelocity=on  PxSenseAcceleration=off  PxSenseTorqueForce=off  PxSenseLowerLimitTorqueForce=off  PxSenseUpperLimitTorqueForce=off  PxLowerLimitSpecify=off  PxLowerLimitBound=-1  PxLowerLimitBoundUnits=m  PxLowerLimitStiffness=1e6  PxLowerLimitStiffnessUnits=N/m  PxLowerLimitDamping=1e3  PxLowerLimitDampingUnits=N/(m/s)  PxLowerLimitTransitionRegionWidth=1e-4  PxLowerLimitTransitionRegionWidthUnits=m  PxUpperLimitSpecify=off  PxUpperLimitBound=1  PxUpperLimitBoundUnits=m  PxUpperLimitStiffness=1e6  PxUpperLimitStiffnessUnits=N/m  PxUpperLimitDamping=1e3  PxUpperLimitDampingUnits=N/(m/s)  PxUpperLimitTransitionRegionWidth=1e-4  PxUpperLimitTransitionRegionWidthUnits=m  PxPositionTargetSpecify=off  PxPositionTargetPriority=High  PxPositionTargetValue=0  PxPositionTargetValueUnits=m  PxVelocityTargetSpecify=off  PxVelocityTargetPriority=High  PxVelocityTargetValue=0  PxVelocityTargetValueUnits=m/s  PyEquilibriumPosition=0  PyEquilibriumPositionUnits=m  PySpringStiffness=0  PySpringStiffnessUnits=N/m  PyDampingCoefficient=1e-3  PyDampingCoefficientUnits=N/(m/s)  PyTorqueActuationMode=NoTorque  PyMotionActuationMode=ComputedMotion  PySensePosition=on  PySenseVelocity=on  PySenseAcceleration=off  PySenseTorqueForce=off  PySenseLowerLimitTorqueForce=off  PySenseUpperLimitTorqueForce=off  PyLowerLimitSpecify=off  PyLowerLimitBound=-1  PyLowerLimitBoundUnits=m  PyLowerLimitStiffness=1e6  PyLowerLimitStiffnessUnits=N/m  PyLowerLimitDamping=1e3  PyLowerLimitDampingUnits=N/(m/s)  PyLowerLimitTransitionRegionWidth=1e-4  PyLowerLimitTransitionRegionWidthUnits=m  PyUpperLimitSpecify=off  PyUpperLimitBound=1  PyUpperLimitBoundUnits=m  PyUpperLimitStiffness=1e6  PyUpperLimitStiffnessUnits=N/m  PyUpperLimitDamping=1e3  PyUpperLimitDampingUnits=N/(m/s)  PyUpperLimitTransitionRegionWidth=1e-4  PyUpperLimitTransitionRegionWidthUnits=m  PyPositionTargetSpecify=off  PyPositionTargetPriority=High  PyPositionTargetValue=0  PyPositionTargetValueUnits=m  PyVelocityTargetSpecify=off  PyVelocityTargetPriority=High  PyVelocityTargetValue=0  PyVelocityTargetValueUnits=m/s  PzEquilibriumPosition=0  PzEquilibriumPositionUnits=m  PzSpringStiffness=0  PzSpringStiffnessUnits=N/m  PzDampingCoefficient=0  PzDampingCoefficientUnits=N/(m/s)  PzTorqueActuationMode=NoTorque  PzMotionActuationMode=ComputedMotion  PzSensePosition=off  PzSenseVelocity=off  PzSenseAcceleration=off  PzSenseTorqueForce=off  PzSenseLowerLimitTorqueForce=off  PzSenseUpperLimitTorqueForce=off  PzLowerLimitSpecify=off  PzLowerLimitBound=-1  PzLowerLimitBoundUnits=m  PzLowerLimitStiffness=1e6  PzLowerLimitStiffnessUnits=N/m  PzLowerLimitDamping=1e3  PzLowerLimitDampingUnits=N/(m/s)  PzLowerLimitTransitionRegionWidth=1e-4  PzLowerLimitTransitionRegionWidthUnits=m  PzUpperLimitSpecify=off  PzUpperLimitBound=1  PzUpperLimitBoundUnits=m  PzUpperLimitStiffness=1e6  PzUpperLimitStiffnessUnits=N/m  PzUpperLimitDamping=1e3  PzUpperLimitDampingUnits=N/(m/s)  PzUpperLimitTransitionRegionWidth=1e-4  PzUpperLimitTransitionRegionWidthUnits=m  PzPositionTargetSpecify=off  PzPositionTargetPriority=High  PzPositionTargetValue=0  PzPositionTargetValueUnits=m  PzVelocityTargetSpecify=off  PzVelocityTargetPriority=High  PzVelocityTargetValue=0  PzVelocityTargetValueUnits=m/s  SphDefPosRotationMethod=None  SphDefPosRotationAngleUnits=deg  SphDefPosRotationStandardAxis=+Z  SphDefPosRotationAngle=0.0  SphDefPosRotationArbitraryAxis=[0 0 1]  SphDefPosFollAlignAxisA=+X  SphDefPosBaseAlignAxisA=+Y  SphDefPosFollAlignAxisB=+Y  SphDefPosBaseAlignAxisB=+Z  SphDefPosRotationSequenceAxes=FollowerAxes  SphDefPosRotationSequence=XYX  SphDefPosRotationSequenceAngles=[0 0 0]  SphDefPosRotationSequenceAnglesUnits=deg  SphDefPosRotationMatrix=[1 0 0; 0 1 0; 0 0 1]  SphEqPosRotationMethod=None  SphEqPosRotationAngleUnits=deg  SphEqPosRotationStandardAxis=+Z  SphEqPosRotationAngle=0.0  SphEqPosRotationArbitraryAxis=[0 0 1]  SphEqPosFollAlignAxisA=+X  SphEqPosBaseAlignAxisA=+Y  SphEqPosFollAlignAxisB=+Y  SphEqPosBaseAlignAxisB=+Z  SphEqPosRotationSequenceAxes=FollowerAxes  SphEqPosRotationSequence=XYX  SphEqPosRotationSequenceAngles=[0 0 0]  SphEqPosRotationSequenceAnglesUnits=deg  SphEqPosRotationMatrix=[1 0 0; 0 1 0; 0 0 1]  SphSpringStiffness=0  SphSpringStiffnessUnits=N*m/deg  SphDampingCoefficient=0  SphDampingCoefficientUnits=N*m/(deg/s)  SphActuateTorqueX=off  SphActuateTorqueY=off  SphActuateTorqueZ=off  SphActuateTorque=off  SphTorqueActuationMode=NoTorque  SphMotionActuationMode=ComputedMotion  SphActuationFrame=BaseFrame  SphSensePosition=off  SphSenseVelocityX=off  SphSenseVelocityY=off  SphSenseVelocityZ=off  SphSenseVelocity=off  SphSenseAccelerationX=off  SphSenseAccelerationY=off  SphSenseAccelerationZ=off  SphSenseAcceleration=off  SphSenseTorqueX=off  SphSenseTorqueY=off  SphSenseTorqueZ=off  SphSenseTorqueForce=off  SphSenseLowerLimitTorqueMag=off  SphSenseUpperLimitTorqueMag=off  SphSensingFrame=BaseFrame  SphLowerLimitSpecify=off  SphLowerLimitBound=15  SphLowerLimitBoundUnits=deg  SphLowerLimitStiffness=1e4  SphLowerLimitStiffnessUnits=N*m/deg  SphLowerLimitDamping=10  SphLowerLimitDampingUnits=N*m/(deg/s)  SphLowerLimitTransitionRegionWidth=0.1  SphLowerLimitTransitionRegionWidthUnits=deg  SphUpperLimitSpecify=off  SphUpperLimitBound=45  SphUpperLimitBoundUnits=deg  SphUpperLimitStiffness=1e4  SphUpperLimitStiffnessUnits=N*m/deg  SphUpperLimitDamping=10  SphUpperLimitDampingUnits=N*m/(deg/s)  SphUpperLimitTransitionRegionWidth=0.1  SphUpperLimitTransitionRegionWidthUnits=deg  SphPositionTargetRotationMethod=None  SphPositionTargetRotationAngleUnits=deg  SphPositionTargetRotationStandardAxis=+Z  SphPositionTargetRotationAngle=0.0  SphPositionTargetRotationArbitraryAxis=[0 0 1]  SphPositionTargetFollAlignAxisA=+X  SphPositionTargetBaseAlignAxisA=+Y  SphPositionTargetFollAlignAxisB=+Y  SphPositionTargetBaseAlignAxisB=+Z  SphPositionTargetRotationSequenceAxes=FollowerAxes  SphPositionTargetRotationSequence=XYX  SphPositionTargetRotationSequenceAngles=[0 0 0]  SphPositionTargetRotationSequenceAnglesUnits=deg  SphPositionTargetRotationMatrix=[1 0 0; 0 1 0; 0 0 1]  SphPositionTargetSpecify=off  SphPositionTargetPriority=High  SphVelocityTargetValue=[0 0 0]  SphVelocityTargetValueUnits=deg/s  SphVelocityTargetSpecify=off  SphVelocityTargetPriority=High  SphVelocityTargetInFollowerFrame=on
  Cartesian Joint : sm_lib/Joints/Cartesian Joint  JointMode=Normal  SenseConstraintForce=off  SenseConstraintForceX=off  SenseConstraintForceY=off  SenseConstraintForceZ=off  SenseConstraintTorque=off  SenseConstraintTorqueX=off  SenseConstraintTorqueY=off  SenseConstraintTorqueZ=off  SenseTotalForce=off  SenseTotalForceX=off  SenseTotalForceY=off  SenseTotalForceZ=off  SenseTotalTorque=off  SenseTotalTorqueX=off  SenseTotalTorqueY=off  SenseTotalTorqueZ=off  CompositeWrenchDir=FollowerOnBase  CompositeWrenchFrame=BaseFrame  PxEquilibriumPosition=0  PxEquilibriumPositionUnits=m  PxSpringStiffness=0  PxSpringStiffnessUnits=N/m  PxDampingCoefficient=1e-3  PxDampingCoefficientUnits=N/(m/s)  PxTorqueActuationMode=NoTorque  PxMotionActuationMode=ComputedMotion  PxSensePosition=on  PxSenseVelocity=on  PxSenseAcceleration=off  PxSenseTorqueForce=off  PxSenseLowerLimitTorqueForce=off  PxSenseUpperLimitTorqueForce=off  PxLowerLimitSpecify=off  PxLowerLimitBound=-1  PxLowerLimitBoundUnits=m  PxLowerLimitStiffness=1e6  PxLowerLimitStiffnessUnits=N/m  PxLowerLimitDamping=1e3  PxLowerLimitDampingUnits=N/(m/s)  PxLowerLimitTransitionRegionWidth=1e-4  PxLowerLimitTransitionRegionWidthUnits=m  PxUpperLimitSpecify=off  PxUpperLimitBound=1  PxUpperLimitBoundUnits=m  PxUpperLimitStiffness=1e6  PxUpperLimitStiffnessUnits=N/m  PxUpperLimitDamping=1e3  PxUpperLimitDampingUnits=N/(m/s)  PxUpperLimitTransitionRegionWidth=1e-4  PxUpperLimitTransitionRegionWidthUnits=m  PxPositionTargetSpecify=off  PxPositionTargetPriority=High  PxPositionTargetValue=0  PxPositionTargetValueUnits=m  PxVelocityTargetSpecify=off  PxVelocityTargetPriority=High  PxVelocityTargetValue=0  PxVelocityTargetValueUnits=m/s  PyEquilibriumPosition=0  PyEquilibriumPositionUnits=m  PySpringStiffness=0  PySpringStiffnessUnits=N/m  PyDampingCoefficient=1e-3  PyDampingCoefficientUnits=N/(m/s)  PyTorqueActuationMode=NoTorque  PyMotionActuationMode=ComputedMotion  PySensePosition=on  PySenseVelocity=on  PySenseAcceleration=off  PySenseTorqueForce=off  PySenseLowerLimitTorqueForce=off  PySenseUpperLimitTorqueForce=off  PyLowerLimitSpecify=off  PyLowerLimitBound=-1  PyLowerLimitBoundUnits=m  PyLowerLimitStiffness=1e6  PyLowerLimitStiffnessUnits=N/m  PyLowerLimitDamping=1e3  PyLowerLimitDampingUnits=N/(m/s)  PyLowerLimitTransitionRegionWidth=1e-4  PyLowerLimitTransitionRegionWidthUnits=m  PyUpperLimitSpecify=off  PyUpperLimitBound=1  PyUpperLimitBoundUnits=m  PyUpperLimitStiffness=1e6  PyUpperLimitStiffnessUnits=N/m  PyUpperLimitDamping=1e3  PyUpperLimitDampingUnits=N/(m/s)  PyUpperLimitTransitionRegionWidth=1e-4  PyUpperLimitTransitionRegionWidthUnits=m  PyPositionTargetSpecify=off  PyPositionTargetPriority=High  PyPositionTargetValue=0  PyPositionTargetValueUnits=m  PyVelocityTargetSpecify=off  PyVelocityTargetPriority=High  PyVelocityTargetValue=0  PyVelocityTargetValueUnits=m/s  PzEquilibriumPosition=0  PzEquilibriumPositionUnits=m  PzSpringStiffness=0  PzSpringStiffnessUnits=N/m  PzDampingCoefficient=0  PzDampingCoefficientUnits=N/(m/s)  PzTorqueActuationMode=NoTorque  PzMotionActuationMode=ComputedMotion  PzSensePosition=off  PzSenseVelocity=off  PzSenseAcceleration=off  PzSenseTorqueForce=off  PzSenseLowerLimitTorqueForce=off  PzSenseUpperLimitTorqueForce=off  PzLowerLimitSpecify=off  PzLowerLimitBound=-1  PzLowerLimitBoundUnits=m  PzLowerLimitStiffness=1e6  PzLowerLimitStiffnessUnits=N/m  PzLowerLimitDamping=1e3  PzLowerLimitDampingUnits=N/(m/s)  PzLowerLimitTransitionRegionWidth=1e-4  PzLowerLimitTransitionRegionWidthUnits=m  PzUpperLimitSpecify=off  PzUpperLimitBound=1  PzUpperLimitBoundUnits=m  PzUpperLimitStiffness=1e6  PzUpperLimitStiffnessUnits=N/m  PzUpperLimitDamping=1e3  PzUpperLimitDampingUnits=N/(m/s)  PzUpperLimitTransitionRegionWidth=1e-4  PzUpperLimitTransitionRegionWidthUnits=m  PzPositionTargetSpecify=off  PzPositionTargetPriority=High  PzPositionTargetValue=0  PzPositionTargetValueUnits=m  PzVelocityTargetSpecify=off  PzVelocityTargetPriority=High  PzVelocityTargetValue=0  PzVelocityTargetValueUnits=m/s
  Chassis : Subsystem
  Gain{,1..3} (4 alike) : Gain  Commented=on
  Gain{4..9} (6 alike) : Gain
  Goto : Goto  Commented=on  GotoTag=x_ref  TagVisibility=global
  Goto1 : Goto  Commented=on  GotoTag=vx_ref  TagVisibility=global
  Goto2 : Goto  Commented=on  GotoTag=y_ref  TagVisibility=global
  Goto3 : Goto  Commented=on  GotoTag=vy_ref  TagVisibility=global
  PS-Simulink Converter{,1..3} (4 alike) : nesl_utility/PS-Simulink Converter  Commented=on  PhysicalDomain=network_engine_domain  SubClassName=ps_output  LeftPortType=input  RightPortType=output  PseudoPeriodic=off  Frequencies=[]  Unit=inherit  AffineConversion=off
      settings: SourceProductBaseCode=PW,SS
  PS-Simulink Converter{4..9} (6 alike) : nesl_utility/PS-Simulink Converter  PhysicalDomain=network_engine_domain  SubClassName=ps_output  LeftPortType=input  RightPortType=output  PseudoPeriodic=off  Frequencies=[]  Unit=inherit  AffineConversion=off
      settings: SourceProductBaseCode=PW,SS
  Revolute Joint : sm_lib/Joints/Revolute Joint  JointMode=Normal  SenseConstraintForce=off  SenseConstraintForceX=off  SenseConstraintForceY=off  SenseConstraintForceZ=off  SenseConstraintTorque=off  SenseConstraintTorqueX=off  SenseConstraintTorqueY=off  SenseConstraintTorqueZ=off  SenseTotalForce=off  SenseTotalForceX=off  SenseTotalForceY=off  SenseTotalForceZ=off  SenseTotalTorque=off  SenseTotalTorqueX=off  SenseTotalTorqueY=off  SenseTotalTorqueZ=off  CompositeWrenchDir=FollowerOnBase  CompositeWrenchFrame=BaseFrame  EquilibriumPosition=0  EquilibriumPositionUnits=deg  SpringStiffness=0  SpringStiffnessUnits=N*m/deg  DampingCoefficient=1e-3  DampingCoefficientUnits=N*m/(deg/s)  TorqueActuationMode=NoTorque  MotionActuationMode=ComputedMotion  SensePosition=on  SenseVelocity=on  SenseAcceleration=off  SenseTorqueForce=off  SenseLowerLimitTorqueForce=off  SenseUpperLimitTorqueForce=off  LowerLimitSpecify=off  LowerLimitBound=-90  LowerLimitBoundUnits=deg  LowerLimitStiffness=1e4  LowerLimitStiffnessUnits=N*m/deg  LowerLimitDamping=10  LowerLimitDampingUnits=N*m/(deg/s)  LowerLimitTransitionRegionWidth=0.1  LowerLimitTransitionRegionWidthUnits=deg  UpperLimitSpecify=off  UpperLimitBound=90  UpperLimitBoundUnits=deg  UpperLimitStiffness=1e4  UpperLimitStiffnessUnits=N*m/deg  UpperLimitDamping=10  UpperLimitDampingUnits=N*m/(deg/s)  UpperLimitTransitionRegionWidth=0.1  UpperLimitTransitionRegionWidthUnits=deg  PositionTargetSpecify=off  PositionTargetPriority=High  PositionTargetValue=0  PositionTargetValueUnits=deg  VelocityTargetSpecify=off  VelocityTargetPriority=High  VelocityTargetValue=0  VelocityTargetValueUnits=deg/s
  Rigid Transform1 : sm_lib/Frames and Transforms/Rigid Transform  TranslationMethod=None  TranslationStandardOffset=0  TranslationLengthUnit=m  TranslationStandardAxis=+Z  TranslationCartesianOffset=[0 0 0]  TranslationROffset=0  TranslationROffsetUnits=m  TranslationZOffset=0  TranslationZOffsetUnits=m  TranslationThetaOffset=0  TranslationThetaOffsetUnits=deg  RotationMethod=StandardAxis  RotationAngleUnits=deg  RotationStandardAxis=+Z  RotationAngle=90  RotationArbitraryAxis=[0 0 1]  FollAlignAxisA=+X  BaseAlignAxisA=+Y  FollAlignAxisB=+Y  BaseAlignAxisB=+Z  RotationSequenceAxes=FollowerAxes  RotationSequence=XYX  RotationSequenceAngles=[0 0 0]  RotationSequenceAnglesUnits=deg  RotationMatrix=[1 0 0; 0 1 0; 0 0 1]
  Wheels : Subsystem  mask{wDamping=wheel.contact.damping, wStiffness=wheel.contact.stiffness, wTransWidth=wheel.contact.transitionRegion, wStatic=wheel.contact.staticFriction, wDynamic=wheel.contact.dynamicFriction, wCritical=wheel.contact.criticalVelocity, TireColor=tire.color, TireDensity=tire.density, TireRadius=tire.radius, wColor=wheel.color, wDensity=wheel.density, wRadius=wheel.radius, wWidth=wheel.width, wAxle=wheel.axleRadius, wResolution=wheel.resolution}
      mask prompts: wDamping "Contact Damping (N/(m/s))"; wStiffness "Contact Stiffness (N/m)"; wTransWidth "Transition Region Width (mm)"; wStatic "Static Friction"; wDynamic "Dynamic Friction"; wCritical "Critical Velocity"; TireColor "Color"; TireDensity "Density (kg/m^3)"; TireRadius "Radius (m)"; wColor "Color"; wDensity "WheelDensity (kg/m^3)"; wRadius "Radius (m)"; wWidth "Width (m)"; wAxle "Axle Radius (m)"; wResolution "Circle Resolution (pts/rev)"
      mask DialogControl WheelContacts Prompt: WheelContacts
      mask DialogControl TabTire Prompt: Tire
      mask DialogControl TireGraphic Prompt: Graphic
      mask DialogControl TireInertia Prompt: Inertia
      mask DialogControl TireGeometry Prompt: Geometry
      mask DialogControl TabWheel Prompt: Wheel
      mask DialogControl WheelGraphic Prompt: Graphic
      mask DialogControl WheelInertia Prompt: Inertia
      mask DialogControl WheelGeometry Prompt: Geometry
  W : PMIOPort  Side=Left
  W1Speed : PMIOPort  Port=2  Side=Left
  W2Speed : PMIOPort  Port=3  Side=Left
  W3Speed : PMIOPort  Port=4  Side=Left
  W4Speed : PMIOPort  Port=5  Side=Left
  Wheels G : PMIOPort  Port=6  Side=Right
  W1_Actual : Outport
  W2_Actual : Outport  Port=2
  W3_Actual : Outport  Port=3
  W4_Actual : Outport  Port=4
  tag scope: vw_ref=global, vx_ref=global, vy_ref=global, w_ref=global, x_ref=global, y_ref=global
  wires:
  Wheels/4(W4_Real) -> W4_Actual/1
  Wheels/1(W3_Real) -> W3_Actual/1
  Wheels/2(W2_Real) -> W2_Actual/1
  Wheels/3(W1_Real) -> W1_Actual/1
  Gain5/1 -> [vw_ref]
  Gain4/1 -> [w_ref]
  Gain3/1 -> Goto3/1
  Gain2/1 -> Goto2/1
  Gain1/1 -> Goto1/1
  Gain/1 -> Goto/1
  PS-Simulink Converter/1 -> Gain/1
  PS-Simulink Converter1/1 -> Gain1/1
  PS-Simulink Converter2/1 -> Gain2/1
  PS-Simulink Converter3/1 -> Gain3/1
  PS-Simulink Converter4/1 -> Gain4/1
  PS-Simulink Converter5/1 -> Gain5/1
  Gain6/1 -> [x_ref]
  PS-Simulink Converter6/1 -> Gain6/1
  Gain8/1 -> [y_ref]
  PS-Simulink Converter9/1 -> Gain9/1
  Gain9/1 -> [vy_ref]
  Gain7/1 -> [vx_ref]
  PS-Simulink Converter8/1 -> Gain8/1
  PS-Simulink Converter7/1 -> Gain7/1
  connections:
  W3Speed/RConn1 -- Wheels/LConn1
  W2Speed/RConn1 -- Wheels/LConn2
  Wheels G/RConn1 -- Wheels/LConn3
  PS-Simulink Converter/LConn1 -- 6-DOF Joint/RConn2
  PS-Simulink Converter1/LConn1 -- 6-DOF Joint/RConn3
  6-DOF Joint/RConn4 -- PS-Simulink Converter2/LConn1
  PS-Simulink Converter3/LConn1 -- 6-DOF Joint/RConn5
  Revolute Joint/RConn3 -- PS-Simulink Converter5/LConn1
  Revolute Joint/RConn2 -- PS-Simulink Converter4/LConn1
  Rigid Transform1/LConn1 -- W/RConn1
  Rigid Transform1/RConn1 -- Revolute Joint/LConn1
  PS-Simulink Converter9/LConn1 -- Cartesian Joint/RConn5
  PS-Simulink Converter8/LConn1 -- Cartesian Joint/RConn4
  PS-Simulink Converter7/LConn1 -- Cartesian Joint/RConn3
  PS-Simulink Converter6/LConn1 -- Cartesian Joint/RConn2
  Chassis/LConn1 -- Cartesian Joint/RConn1
  Revolute Joint/RConn1 -- Cartesian Joint/LConn1
  W1Speed/RConn1 -- Wheels/LConn4
  W4Speed/RConn1 -- Wheels/LConn5
  Wheels/RConn4 -- Chassis/LConn5
  Chassis/LConn2 -- Wheels/RConn3
  Chassis/LConn3 -- Wheels/RConn2
  Wheels/RConn1 -- Chassis/LConn4

== system robot_simplified/Subsystem ==
  IsRef : Inport
  Is : Inport  Port=2
  Reset : Inport  Port=3
  Hall : Inport  Port=4
  Direction : Inport  Port=5
  BLDC Current Controller with PWM Generation : eeBldcCurrentController/BLDC Current Controller with PWM Generation  Kp=1  Ki=5  Kaw=1  Ts=-1  Tsd=0.001  ActZC=off  CarrCount=Up  Tper=0.001  Tfundamental=0.0001
      settings: SourceProductBaseCode=PS
  G : Outport
  wires:
  BLDC Current Controller with PWM Generation/1 -> G/1
  Is/1 -> BLDC Current Controller with PWM Generation/2
  Direction/1 -> BLDC Current Controller with PWM Generation/5
  Hall/1 -> BLDC Current Controller with PWM Generation/4
  Reset/1 -> BLDC Current Controller with PWM Generation/3
  IsRef/1 -> BLDC Current Controller with PWM Generation/1
